simulink model "washing_machine_stateflow"  (R2024b)
settings: Solver=VariableStepAuto  StartTime=0.0  StopTime=inf  RelTol=1e-3
settings Model: Creator=KHALID  LastModifiedBy=KHALID

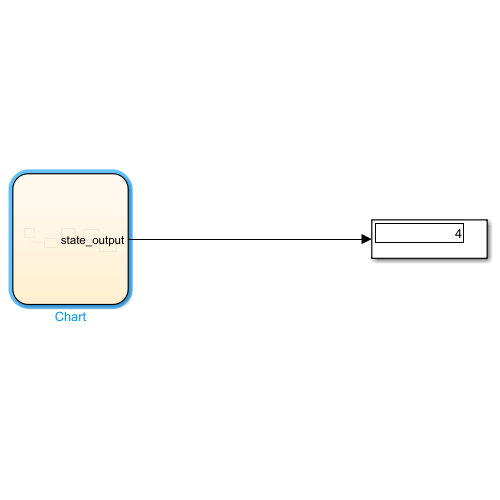
[thumbnail: Simulink's stored preview of the top-level diagram]
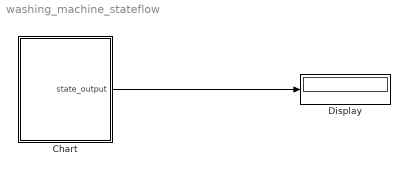
== system washing_machine_stateflow ==
  Chart : Stateflow chart  TreatAsAtomicUnit=on
  Display : Display
  wires:
  Chart/1(state_output) -> Display/1

== stateflow chart washing_machine_stateflow/Chart ==
  state Rinse
    entry:disp('Rinsing clothes...');
    after(3,sec);
    state_output=3;
  state Fill
    entry:disp('Filling water ..');
    after(3,sec);
    state_output=1;
  state Spin
    entry:disp('Spinning Clothes....');
    after(3,sec);
    state_output=4;
  state Wash
    entry:disp('Washing clothes...');
    after(3,sec);
    state_output=2;
  state Complete
    entry:disp('Washing Cycle is completed');
    after(3,sec);
    state_output=5;
  (default) -> Fill : {state_output=0}
  Rinse -> Spin : [state_output==3&&after(5,sec)]
  Spin -> Complete : [state_output==4&&after(5,sec)]
  Fill -> Wash : [state_output==1&&after(5,sec)]
  Wash -> Rinse : [state_output==2&&after(5,sec)]
  data: state_output output
